simulink model "beta5al1_5_v"  (R2019b)
settings: Solver=ode4  StartTime=0.0  StopTime=6e6  FixedStep=1  RelTol=1e-3
values from neighbouring files (symbols this model uses):
  dataT = dataTT(r)    [CCspeed.m]
libraries: simulink x1
settings Model: Creator=Administrator  LastModifiedBy=User
settings DataIOCC: ReturnWorkspaceOutputs=off
settings OptimizationCC: LifeSpan=inf
settings DebuggingCC: AlgebraicLoopMsg=none  SFExecutionAtInitializationDiag=none  ArithmeticOperatorsInVariantConditions=warning
settings SFSimCC: SimUseLocalCustomCode=off  CustomCodeUndefinedFunction=UseInterfaceOnly
settings RTWCC: RTWUseLocalCustomCode=off
settings CodeAppCC: StateflowObjectComments=on

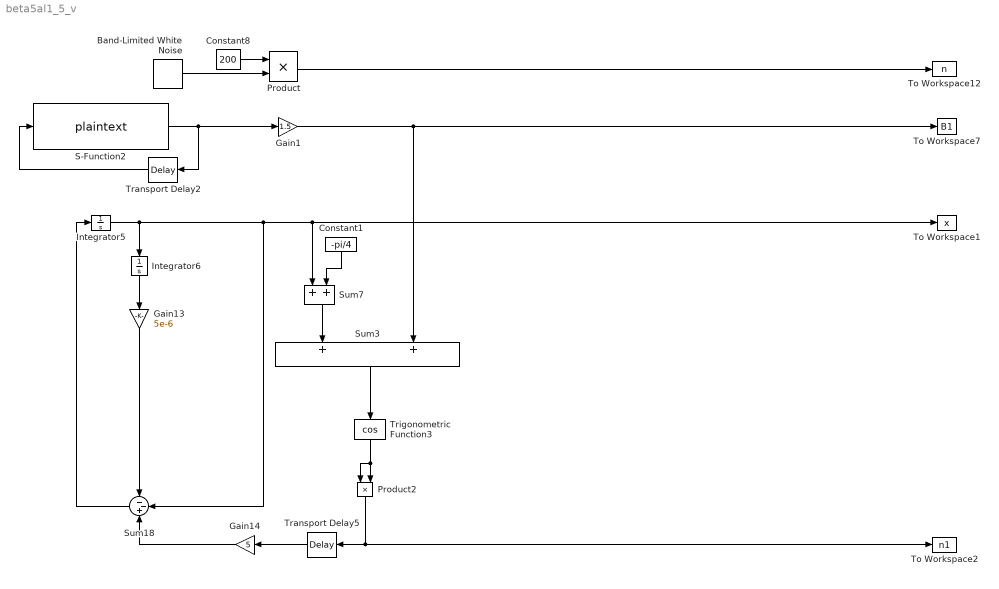
== system beta5al1_5_v ==
  Band-Limited White Noise : simulink/Sources/Band-Limited White Noise  Cov=[0.0000001]  Ts=1  seed=[23341]
  Constant1 : Constant  Value=-pi/4
  Constant8 : Constant  Value=200
  Gain1 : Gain  Gain=1.5
  Gain13 : Gain  Gain=5e-6
  Gain14 : Gain  Gain=5
  Integrator5 : Integrator  InitialCondition=0.1
  Integrator6 : Integrator
  Product : Product
  Product2 : Product
  S-Function2 : S-Function  FunctionName=plaintext  Parameters=dataT,1  SFunctionDeploymentMode=off  EnableBusSupport=off
  Sum18 : Sum  Inputs=--+
  Sum3 : Sum
  Sum7 : Sum
  To Workspace1 : ToWorkspace  VariableName=x  SampleTime=-1
  To Workspace12 : ToWorkspace  VariableName=n  SampleTime=-1
  To Workspace2 : ToWorkspace  VariableName=n1  SampleTime=-1
  To Workspace7 : ToWorkspace  VariableName=B1  SampleTime=-1
  Transport Delay2 : TransportDelay
  Transport Delay5 : TransportDelay  DelayTime=1200  BufferSize=100000
  Trigonometric Function3 : Trigonometry  Operator=cos  OutputSignalType=real
  wires:
  Trigonometric Function3/1 -> Product2/1, Product2/2
  Integrator5/1 -> Sum18/2, Sum7/1, To Workspace1/1, Integrator6/1
  Gain13/1 -> Sum18/1
  Transport Delay5/1 -> Gain14/1
  Integrator6/1 -> Gain13/1
  Sum18/1 -> Integrator5/1
  Constant1/1 -> Sum7/2
  Transport Delay2/1 -> S-Function2/1
  S-Function2/1 -> Transport Delay2/1, Gain1/1
  Constant8/1 -> Product/1
  Product/1 -> To Workspace12/1
  Band-Limited White Noise/1 -> Product/2
  Gain14/1 -> Sum18/3
  Sum7/1 -> Sum3/1
  Sum3/1 -> Trigonometric Function3/1
  Product2/1 -> To Workspace2/1, Transport Delay5/1
  Gain1/1 -> To Workspace7/1, Sum3/2
